simulink model "abe_slope_limiter"  (R2022a)
settings: Solver=VariableStepAuto  StartTime=0.0  StopTime=50  RelTol=1e-3
libraries: simulink x1
settings Model: Creator=Abraham  LastModifiedBy=Abraham

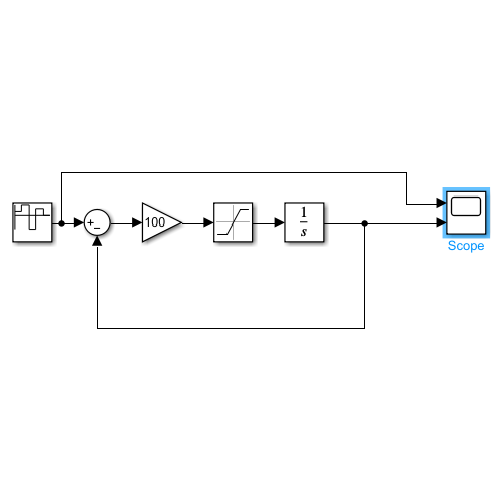
[thumbnail: Simulink's stored preview of the top-level diagram]
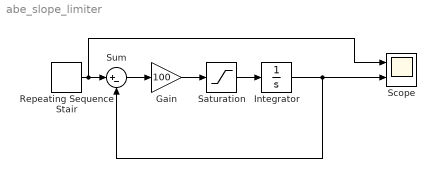
== system abe_slope_limiter ==
  Gain : Gain  Gain=100
  Integrator : Integrator
  Repeating Sequence Stair : simulink/Sources/Repeating Sequence Stair  OutValues=[5 15 -20 10 0]  tsamp=10  OutMin=[]  OutMax=[]  OutDataTypeStr=double  OutputDataTypeScalingMode=double  OutDataType=fixdt(0,8)  ConRadixGroup=Best Precision: Vector-wise  OutScaling=2^-12
  Saturation : Saturate  UpperLimit=10  LowerLimit=-10
  Scope : Scope  NumInputPorts=2
  Sum : Sum  Inputs=|+-
  wires:
  Gain/1 -> Saturation/1
  Saturation/1 -> Integrator/1
  Repeating Sequence Stair/1 -> Scope/1, Sum/1
  Sum/1 -> Gain/1
  Integrator/1 -> Scope/2, Sum/2
